simulink model "motor_test_arm"  (R2017a)
settings: Solver=FixedStepDiscrete  StartTime=0.0  StopTime=inf  RelTol=1e-3
PostLoadFcn:
  | PWMFreq = 400;  % 2500ms period
  | Ts = 1/5e3;
undefined symbols (not defined in the file or in its folder): AXI4, Lite
libraries: axiinterfacelib x3
settings Model: ExtModeTrigDuration=100  Creator=skuznick  LastModifiedBy=skuznick
settings DataIOCC: LimitDataPoints=on  SaveFormat=Array  SaveOutput=off  SaveTime=off
settings OptimizationCC: BlockReduction=off  ConditionallyExecuteInputs=off  LifeSpan=Inf  MaxStackSize=64
settings DebuggingCC: AlgebraicLoopMsg=error  UnderspecifiedInitializationDetection=Classic  MergeDetectMultiDrivingBlocksExec=none  SingleTaskRateTransMsg=error  StrictBusMsg=ErrorOnBusTreatedAsVector  SFUnexpectedBacktrackingDiag=warning  SFNoUnconditionalDefaultTransitionDiag=warning  SFExecutionAtInitializationDiag=none
settings HardwareCC: ProdBitPerPointer=32  ProdBitPerSizeT=32  ProdBitPerPtrDiffT=32  ProdLargestAtomicInteger=Long  ProdLargestAtomicFloat=Double  ProdIntDivRoundTo=Undefined  ProdWordSize=32  ProdHWDeviceType=ARM Compatible->ARM Cortex  ProdEqTarget=off
settings ModelReferenceCC: PropagateSignalLabelsOutOfModel=off
settings SFSimCC: MATLABDynamicMemAlloc=off
settings RTWCC: SystemTargetFile=ert.tlc  HardwareBoard=ZedBoard  TLCOptions=-aInlineSetEventsForThisBaseRateFcn=TLC_FALSE -aSuppressMultiTaskScheduler=TLC_FALSE -aRateBasedStepFcn=0  TemplateMakefile=ert_default_tmf  Description=Embedded Coder  RTWVerbose=off  Toolchain=Xilinx Software Development Kit (SDK)
settings CodeAppCC: IgnoreCustomStorageClasses=off
settings ERTTargetCC: MultiwordLength=2048  ConvertIfToSwitch=off  SuppressUnreachableDefaultCases=off
settings ConfigComp: CovMetricSettings=dw  CovHtmlReporting=on  CovSaveCumulativeToWorkspaceVar=on  CovSaveSingleToWorkspaceVar=on  CovExternalEMLEnable=off

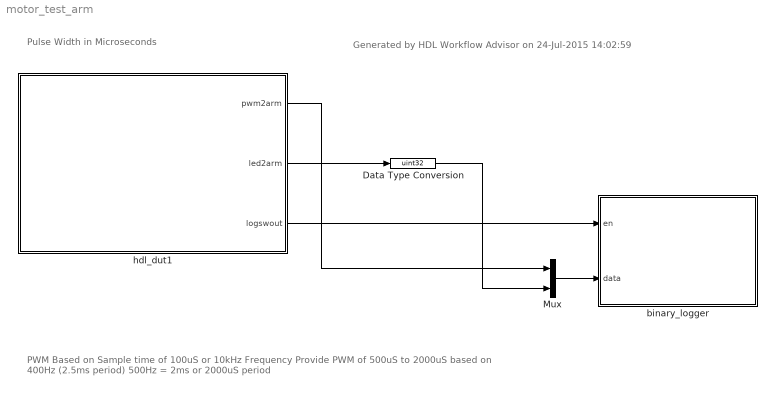
== system motor_test_arm ==
  note: PWM Based on Sample time of 100uS or 10kHz Frequency
      | Provide PWM of 500uS to 2000uS based on 400Hz (2.5ms period)
      | 500Hz = 2ms or 2000uS period
  note: Pulse Width in Microseconds
  note: Generated by HDL Workflow Advisor on 24-Jul-2015 14:02:59
  Data Type Conversion : DataTypeConversion  OutDataTypeStr=uint32
  Mux : Mux  Inputs=2
  binary_logger : MATLAB Function  TreatAsAtomicUnit=on  mask(Pixhawk Binary Logger){logfile=/mnt/datalog}
      mask prompts: logfile "Log File Name Prefix"
      mask help: Log a vector of double data to a file on the SD card
      mask init:
      | logname=uint8(logfile);
  hdl_dut1 : Subsystem  TreatAsAtomicUnit=on  mask(AXI4-Lite/AXI4 Interface){fpgaClk=50e6}
      mask prompts: fpgaClk "FPGA System Clock Freq"
      mask help:
      | This is an automatically generated subsystem block.
      | This contains the AXI interface blocks that communicate with the pwm_ipcore IPCore generated from motor_test/hdl_dut subsystem.
      mask Display: disp(sprintf('Xilinx Zynq \nAXI Interface'));
  wires:
  hdl_dut1/2(led2arm) -> Data Type Conversion/1
  hdl_dut1/3(logswout) -> binary_logger/1(en)
  hdl_dut1/1(pwm2arm) -> Mux/1
  Mux/1 -> binary_logger/2(data)
  Data Type Conversion/1 -> Mux/2

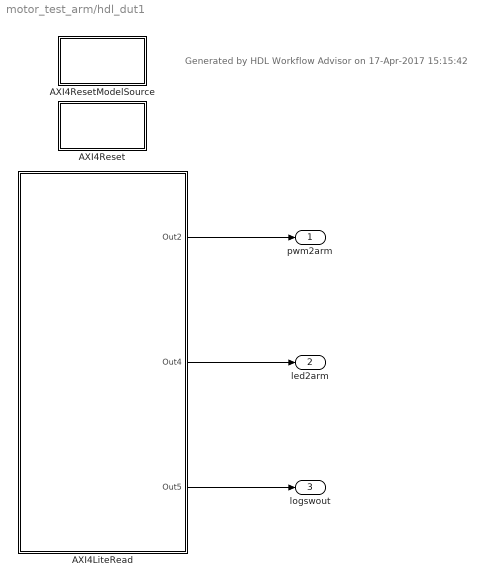
== system motor_test_arm/hdl_dut1 ==
  note: Generated by HDL Workflow Advisor on 17-Apr-2017 15:15:42
  AXI4LiteRead : Subsystem  Priority=10
  AXI4Reset : Subsystem  mask(System Start){ShowInLibBrowser=0}
      mask prompts: ShowInLibBrowser "Simulink:masks:CustCodeMaskParam1_MP"
      settings: CopyFcn=cccopyfcn(gcb)  OpenFcn=ccopenfcn('System Start Function')
      mask Help: eval('feval(''rtwprivate'',''rtwhelpview'',''rtw_sys_start_block'')');
      mask Display: disp('System\nStart');
  AXI4ResetModelSource : Subsystem  mask(Model Source){ShowInLibBrowser=0}
      mask prompts: ShowInLibBrowser "Simulink:masks:CustCodeMaskParam1_MP"
      settings: CopyFcn=cccopyfcn(gcb)  OpenFcn=ccopenfcn('Model Source')
      mask Help: eval('feval(''rtwprivate'',''rtwhelpview'',''rtw_model_source_block'')');
      mask Display: disp('Model\nSource');
  pwm2arm : Outport
  led2arm : Outport  Port=2
  logswout : Outport  Port=3
  wires:
  AXI4LiteRead/1(Out2) -> pwm2arm/1
  AXI4LiteRead/2(Out4) -> led2arm/1
  AXI4LiteRead/3(Out5) -> logswout/1

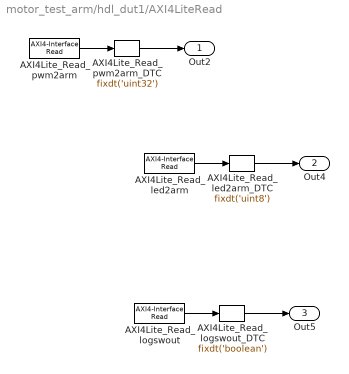
== system motor_test_arm/hdl_dut1/AXI4LiteRead ==
  AXI4Lite_Read_led2arm : axiinterfacelib/AXI4-Interface Read  Priority=5  AXIInterfaceType=AXI4-Lite  DeviceName=/dev/mwipcore  RegisterOffset=hex2dec('104')  DataLength=1  DataType=uint32  SampleTime=-1  blockPlatform=ZYNQ  SimulateUsing=Interpreted Execution
      settings: SourceProductName=Embedded Coder Support Package for Xilinx Zynq-7000 Platform  SourceProductBaseCode=ECZYNQ7000
  AXI4Lite_Read_led2arm_DTC : DataTypeConversion  OutDataTypeStr=fixdt('uint8')  ConvertRealWorld=Stored Integer (SI)
  AXI4Lite_Read_logswout : axiinterfacelib/AXI4-Interface Read  Priority=6  AXIInterfaceType=AXI4-Lite  DeviceName=/dev/mwipcore  RegisterOffset=hex2dec('108')  DataLength=1  DataType=uint32  SampleTime=-1  blockPlatform=ZYNQ  SimulateUsing=Interpreted Execution
      settings: SourceProductName=Embedded Coder Support Package for Xilinx Zynq-7000 Platform  SourceProductBaseCode=ECZYNQ7000
  AXI4Lite_Read_logswout_DTC : DataTypeConversion  OutDataTypeStr=fixdt('boolean')  ConvertRealWorld=Stored Integer (SI)
  AXI4Lite_Read_pwm2arm : axiinterfacelib/AXI4-Interface Read  Priority=4  AXIInterfaceType=AXI4-Lite  DeviceName=/dev/mwipcore  RegisterOffset=hex2dec('100')  DataLength=1  DataType=uint32  SampleTime=-1  blockPlatform=ZYNQ  SimulateUsing=Interpreted Execution
      settings: SourceProductName=Embedded Coder Support Package for Xilinx Zynq-7000 Platform  SourceProductBaseCode=ECZYNQ7000
  AXI4Lite_Read_pwm2arm_DTC : DataTypeConversion  OutDataTypeStr=fixdt('uint32')  ConvertRealWorld=Stored Integer (SI)
  Out2 : Outport
  Out4 : Outport  Port=2
  Out5 : Outport  Port=3
  wires:
  AXI4Lite_Read_led2arm/1 -> AXI4Lite_Read_led2arm_DTC/1
  AXI4Lite_Read_led2arm_DTC/1 -> Out4/1
  AXI4Lite_Read_logswout_DTC/1 -> Out5/1
  AXI4Lite_Read_logswout/1 -> AXI4Lite_Read_logswout_DTC/1
  AXI4Lite_Read_pwm2arm/1 -> AXI4Lite_Read_pwm2arm_DTC/1
  AXI4Lite_Read_pwm2arm_DTC/1 -> Out2/1

== system motor_test_arm/hdl_dut1/AXI4Reset ==

== system motor_test_arm/hdl_dut1/AXI4ResetModelSource ==

== matlab function motor_test_arm/binary_logger ==
  data: en input boolean; data input; logname parameter uint8
%% Binary Logger
% Note: All data needs to be of the same type (e.g. double)
% Header information format:
%           String "MWLOGV##"
%           Time/Date 4 bytes (time())
%           Number of Signals per record Logged 1 byte (256 max)
%           Data Type of Signals Logged  1 byte (1-10)
%           Number of bytes per record 2 bytes (65535 max)
% This does NOT include the number of data sets logged.  
% i.e. The Reader is responsible for reading until EOF.
% MathWorks Pilot Engineering 2015
% Steve Kuznicki
function binary_logger(en, data, logname)
%#codegen

    coder.cinclude('<stdio.h>');
    coder.cinclude('<time.h>');
    persistent fp isflushed isopen count lognumstr

    if isempty(count)
        count = 0;
        lognumstr = 65;
        isopen = false;
        fp = coder.opaque('FILE*', 'NULL');
        isflushed = false;
    end
    
    [elsize, eltype] = get_elem_size(data);
    elem_size = coder.const(uint16(elsize));
    elem_type = coder.const(uint8(eltype));
    vect_size = coder.const(uint8(numel(data)));
    
    if (en)
        if isopen == false
            fp = coder.ceval('fopen', [logname, '_', char(lognumstr), '.bin', int8(0)], ['wb', int8(0)]);
            lognumstr = lognumstr + 1;
            isflushed = false;
            isopen = true;
            % Write header information here
            % header token + version
            mlStrVer = 'MWLOGV01';
            coder.ceval('fwrite', coder.rref(mlStrVer), 1, length(mlStrVer), fp);
            % date/time
            tm = uint32(0);
            tmptr = uint32(0);
            tm = coder.ceval('time',coder.wref(tmptr));
            coder.ceval('fwrite', coder.rref(tm), 4, 1, fp);
            % number of elements in each record
            coder.ceval('fwrite', coder.rref(vect_size), 1, 1, fp);
            % data type of the elements
            coder.ceval('fwrite', coder.rref(elem_type), 1, 1, fp);
            % size of each record in bytes
            recSize = elem_size * uint16(vect_size);
            coder.ceval('fwrite', coder.rref(recSize), 2, 1, fp);
        end
        coder.ceval('fwrite', coder.rref(data), elem_size, vect_size, fp);
        count = count + 1;
        if count >= 100
            coder.ceval('fflush', fp);
            isflushed = false;
            count = 0;
        end
    else
        if ~isflushed
            coder.ceval('fflush', fp);
            isflushed = true;
        end
        coder.ceval('fclose', fp);
        isopen = false;
    end
end

% return the size of the element in bytes
function [elem_size, dtype] = get_elem_size(data)
    switch(class(data))
        case 'double'
            elem_size = 8;
            dtype = 1;
        case 'single'
            elem_size = 4;
            dtype = 2;
        case 'int32'
            elem_size = 4;
            dtype = 3;
        case 'uint32'
            elem_size = 4;
            dtype = 4;
        case 'int16'
            elem_size = 2;
            dtype = 5;
        case 'uint16'
            elem_size = 2;
            dtype = 6;
        case 'int8'
            elem_size = 1;
            dtype = 7;
        case 'uint8'
            elem_size = 1;
            dtype = 8;
        case 'logical'
            elem_size = 1;
            dtype = 9;
        case 'embedded.fi'
            nt = numerictype(data);
            elem_size = 2^ceil(log2(ceil(nt.WordLength / 8)));
            dtype = 10;
    end
    if ~isreal(data)
        elem_size = elem_size*2;
    end
    
    elem_size = uint16(elem_size);
    dtype = uint8(dtype);
end
